simulink model "distance_to_bounding_box"  (R2018a)
settings: Solver=VariableStepAuto  StartTime=0.0  StopTime=10.0  RelTol=1e-3
settings Model: Creator=blond  LastModifiedBy=blond

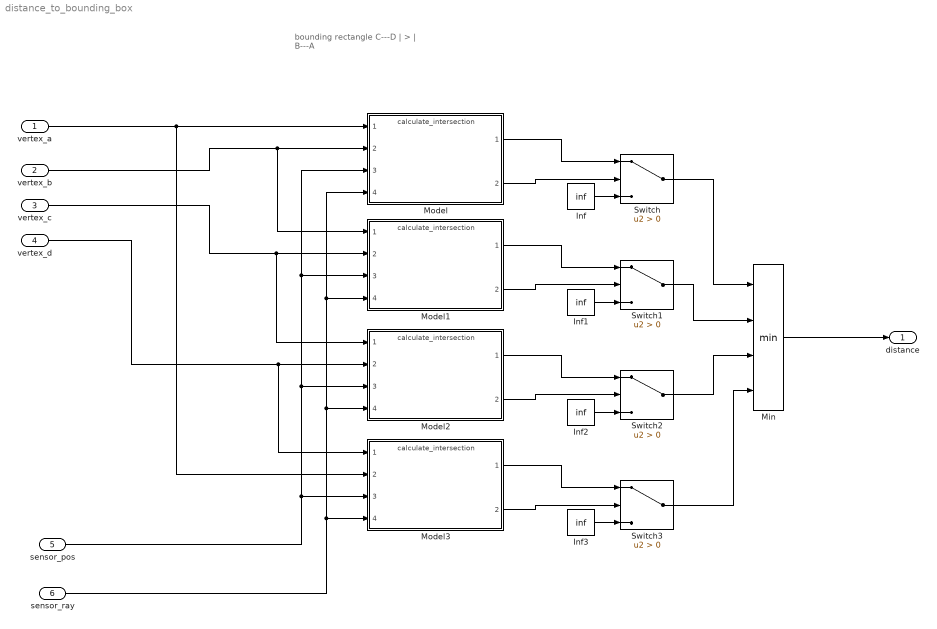
== system distance_to_bounding_box ==
  note: bounding rectangle
      | C---D
      | |  >  |
      | B---A
  "vertex_a " : Inport
  vertex_b : Inport  Port=2
  vertex_c : Inport  Port=3
  vertex_d : Inport  Port=4
  sensor_pos : Inport  Port=5
  "sensor_ray " : Inport  Port=6
  Inf{,1..3} (4 alike) : Constant  Value=inf
  Min : MinMax  Inputs=4  ZeroCross=off
  Model{,1..3} (4 alike) : ModelReference  ModelNameDialog=calculate_intersection.slx  SimulationMode=Normal  ModelReferenceVersion=1.4
  Switch{,1..3} (4 alike) : Switch  Criteria=u2 > Threshold
  distance : Outport
  wires:
  Model1/2 -> Switch1/2
  Model2/2 -> Switch2/2
  Model3/2 -> Switch3/2
  Model3/1 -> Switch3/1
  Switch3/1 -> Min/4
  Inf1/1 -> Switch1/3
  Switch2/1 -> Min/3
  Switch1/1 -> Min/2
  vertex_b/1 -> Model1/1, Model/2
  Switch/1 -> Min/1
  Inf/1 -> Switch/3
  sensor_pos/1 -> Model3/3, Model2/3, Model1/3, Model/3
  "sensor_ray "/1 -> Model3/4, Model2/4, Model1/4, Model/4
  "vertex_a "/1 -> Model3/2, Model/1
  vertex_c/1 -> Model2/1, Model1/2
  Inf2/1 -> Switch2/3
  Model/2 -> Switch/2
  Model1/1 -> Switch1/1
  Inf3/1 -> Switch3/3
  Min/1 -> distance/1
  Model/1 -> Switch/1
  vertex_d/1 -> Model3/1, Model2/2
  Model2/1 -> Switch2/1
